simulink model "sf_matrix"  (Simulink 6.0)
settings: Solver=ode45  StartTime=0.0  StopTime=1  MaxStep=1  RelTol=1e-3
settings Model: CovMetricSettings=dcmtr  Creator=The MathWorks Inc.  LastModifiedBy=batserve  ExtModeAutoUpdateStatusClock=off
settings OptimizationCC: BooleanDataType=off
settings DebuggingCC: CheckExecutionContextPreStartOutputMsg=on  CheckExecutionContextRuntimeOutputMsg=on  SolverPrmCheckMsg=none
settings HardwareCC: TargetUnknown=on

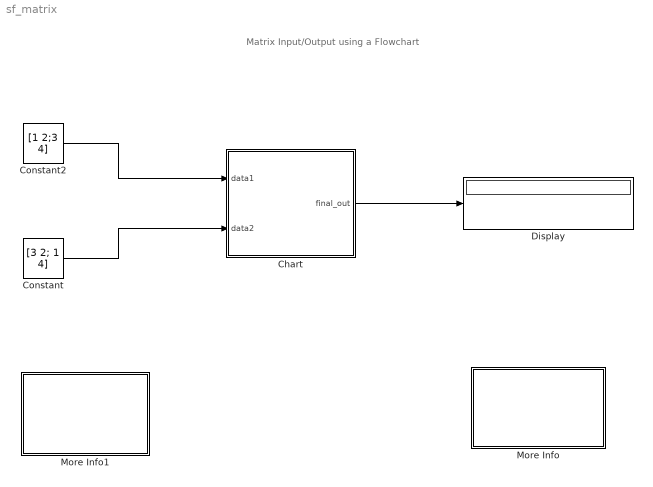
== system sf_matrix ==
  note: Matrix Input/Output using a Flowchart
  Chart : Stateflow chart  PropExecContextAcrossSSBoundary=on
  Constant : Constant  Value=[3 2; 1 4]  VectorParams1D=off
  Constant2 : Constant  Value=[1 2;3 4]  VectorParams1D=off
  Display : Display
  More Info : Subsystem  PropExecContextAcrossSSBoundary=on
      mask Display: disp('Double click\nhere for\ninformation on\nthis demonstration')
  More Info1 : Subsystem  PropExecContextAcrossSSBoundary=on
      settings: OpenFcn=simcad(bdroot);
      mask Display: disp('Double click\nhere for\nSimulink\Stateflow\n Help')
  wires:
  Constant2/1 -> Chart/1(data1)
  Constant/1 -> Chart/2(data2)
  Chart/1(final_out) -> Display/1

== system sf_matrix/More Info ==
  note: Matrix Input/Output Demonstration
  note: The demo illustrates the ability of Stateflow to accept matrix input signals from Simulink and also
      | output matrix signals to Simulink. In this particular example, we are multiplying a [2x2] matrix with another
      | [2x2] matrix to obtain a [2x2] output matrix. A flow chart is used to perform the calculations which is
      | also the reason why the length of the simulation time is only one timestep.
      |
      | The graphical flowchart is equivalent to writing the following nested-loop in the C language:
      |
      | for(i=0;i<2;i++)
      |    for(j=0;j<2;j++)
      |        {
      |          int final_out[2][2];
      |          final_out[i][j]=(data1[i][0]*data2[0][j])+(data1[i][1]+data2[1][j]);
      |        }
      |
      |
      | 'final_out' would be the output Simulink in this demo.

== system sf_matrix/More Info1 ==

== stateflow chart Chart ==
  note: Equivalent C-Code:
      |
      | for(i=0;i<2;i++)
      |    for(j=0;j<2;j++)
      |        {
      |          int final_out[2][2];
      |          final_out[i][j]=(data1[i][0]*data2[0][j])+(data1[i][1]+data2[1][j]);
      |        }
  (default) -> (junction 4) : {final_out[0][0]=(data1[0][0]*data2[0][0])+(data1[0][1]*data2[1][0]);}
  (junction 4) -> (junction 5) : {final_out[0][1]=(data1[0][0]*data2[0][1])+(data1[0][1]*data2[1][1]);}
  (junction 5) -> (junction 6) : {final_out[1][0]=(data1[1][0]*data2[0][0])+(data1[1][1]*data2[1][0]);}
  (junction 6) -> (junction 7) : {final_out[1][1]=(data1[1][0]*data2[0][1])+(data1[1][1]*data2[1][1]);}
  (junction 7) -> (junction 8)
  data: final_out output double size=[2 2]; data1 input double size=[2 2]; data2 input double size=[2 2]
